simulink model "Lookup"  (R2020a)
settings: Solver=FixedStepDiscrete  StartTime=0.0  StopTime=8  FixedStep=1.0  RelTol=1e-3
undefined symbols (not defined in the file or in its folder): Var1, Var2
libraries: simulink x2
settings Model: Creator=hussein  LastModifiedBy=hussein

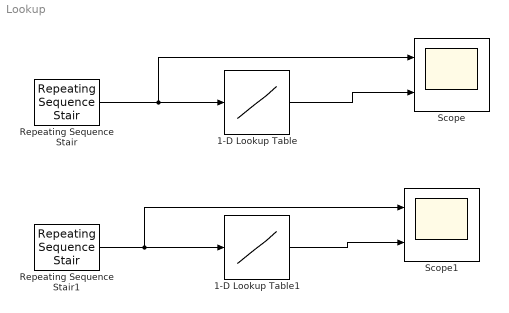
== system Lookup ==
  1-D Lookup Table : Lookup_n-D  NumberOfTableDimensions=1  BreakpointsForDimension1=[0.5:0.04:4.5]  Table=[0:1:100]  InternalRulePriority=Speed  RndMeth=Simplest  InputSameDT=on
  1-D Lookup Table1 : Lookup_n-D  NumberOfTableDimensions=1  BreakpointsForDimension1=Var1  Table=Var2  InternalRulePriority=Speed  RndMeth=Simplest  InputSameDT=on
  Repeating Sequence Stair : simulink/Sources/Repeating Sequence Stair  OutValues=SensorData  tsamp=-1  OutMin=[]  OutMax=[]  OutDataTypeStr=double  OutputDataTypeScalingMode=double  OutDataType=fixdt(0,8)  ConRadixGroup=Best Precision: Vector-wise  OutScaling=2^-12
  Repeating Sequence Stair1 : simulink/Sources/Repeating Sequence Stair  OutValues=[0.5 0.9 1.4 1.8 2.5 4.2 3.7].'  tsamp=-1  OutMin=[]  OutMax=[]  OutDataTypeStr=double  OutputDataTypeScalingMode=double  OutDataType=fixdt(0,8)  ConRadixGroup=Best Precision: Vector-wise  OutScaling=2^-12
  Scope : Scope  NumInputPorts=2
  Scope1 : Scope  NumInputPorts=2
  wires:
  Repeating Sequence Stair/1 -> Scope/1, 1-D Lookup Table/1
  Repeating Sequence Stair1/1 -> Scope1/1, 1-D Lookup Table1/1
  1-D Lookup Table/1 -> Scope/2
  1-D Lookup Table1/1 -> Scope1/2
